simulink model "larix2_tuner"  (R2020b)
settings: Solver=FixedStepDiscrete  StartTime=0.0  StopTime=6  FixedStep=0.002  RelTol=1e-3
PostLoadFcn:
  | load('ThrustTable.mat');
  | init();
values from neighbouring files (symbols this model uses):
  g = 9.810    (= 9.81)    [init.m]
undefined symbols (not defined in the file or in its folder): DiscIntNeverNeededParam
libraries: slpidlib x9, sharedtransform x2, aerolibutil x1
settings Model: Creator=ac114611  LastModifiedBy=wendelin
settings DataIOCC: ExternalInput=getinputstruct(op_hover)  InitialState=getstatestruct(op_hover)  LoadExternalInput=on  LoadInitialState=on  ReturnWorkspaceOutputs=off
settings OptimizationCC: DefaultParameterBehavior=Inlined  EnhancedBackFolding=on  PassReuseOutputArgsAs=Individual arguments  MaxStackSize=64  OptimizeBlockOrder=speed  DifferentSizesBufferReuse=on  EfficientTunableParamExpr=on
settings DebuggingCC: ParameterPrecisionLossMsg=none  ParameterTunabilityLossMsg=error  ArithmeticOperatorsInVariantConditions=warning
settings HardwareCC: ProdBitPerPointer=32  ProdBitPerSizeT=32  ProdBitPerPtrDiffT=32  ProdLargestAtomicInteger=Long  ProdLargestAtomicFloat=Double  ProdWordSize=32  ProdHWDeviceType=ARM Compatible->ARM Cortex  TargetBitPerLong=64  TargetBitPerPointer=64  TargetBitPerSizeT=64  TargetBitPerPtrDiffT=64  TargetLongLongMode=on  TargetIntDivRoundTo=Zero  TargetEndianess=LittleEndian  TargetWordSize=64  TargetHWDeviceType=MATLAB Host  ProdEqTarget=off
settings SFSimCC: SimUseLocalCustomCode=off  MATLABDynamicMemAlloc=off  CustomCodeUndefinedFunction=UseInterfaceOnly
settings RTWCC: Description=Embedded Coder  SystemTargetFile=ert.tlc  GenCodeOnly=on  PackageName=larix2_codegen.zip  TemplateMakefile=ert_default_tmf  RTWUseLocalCustomCode=off  Toolchain=GNU gcc/g++ | gmake (64-bit Linux)  IncludeHyperlinkInReport=on  GenerateCodeMetricsReport=on
settings CodeAppCC: ForceParamTrailComments=on  IgnoreCustomStorageClasses=off  OperatorAnnotations=on  SimulinkDataObjDesc=on  SFDataObjDesc=on  InsertBlockDesc=on
settings ERTTargetCC: TargetLangStandard=C99 (ISO)  InlinedParameterPlacement=NonHierarchical  ERTCustomFileTemplate=example_file_process.tlc

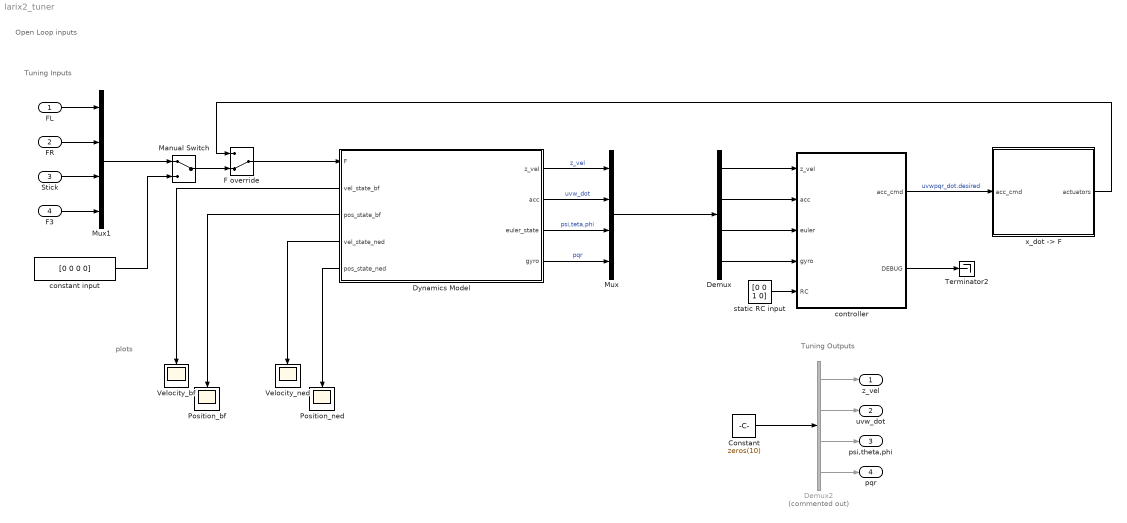
== system larix2_tuner ==
  note: Open Loop inputs
  note: plots
  note: Tuning Inputs
  note: Tuning Outputs
  FL : Inport  PortDimensions=1
  FR : Inport  Port=2
  Stick : Inport  Port=3
  F3 : Inport  Port=4
  Constant : Constant  Value=zeros(10)
  Demux : Demux
  Demux2 : Demux  Commented=on
  Dynamics Model : Subsystem
      settings: PortSchema="{\"entries\":[{\"content\":{\"sides\":[{\"content\":{\"connectorIds\":[\"In1\",\"Out5\",\"Out6\",\"Out7\",\"Out8\"]},\"type\":\"ConnectorPlacement.EquallySpacedRectSide\",\"uuid\":\"7b482eda-451f-4705-a72e-674db1e2ea8f\"},{\"content\":{\"connectorIds\":[\"Out1\",\"Out2\",\"Out3\",\"Out4\"],\"side\":\"RIGHT\"},\"type\":\"ConnectorPlacement.EquallySpacedRectSide\",\"uuid\":\"2344d3e9-2a2c-4bd3-8790-1f9d37abcd4c\"},{\"content\":{\"connectorIds\":[],\"side\":\"TOP\"},\"type\":\"ConnectorPlacement.EquallySpacedRectSide\",\"uuid\":\"13a22bb4-0a82-4477-a366-02f381e5ef07\"},{\"content\":{\"connectorIds\":[],\"side\":\"BOTTOM\"},\"type\":\"ConnectorPlacement.EquallySpacedRectSide\",\"uuid\":\"663825dc-fe4c-484f-87e0-eae3c1c76089\"},{\"content\":{\"connectorIds\":[],\"side\":\"HIDDEN\"},\"type\":\"ConnectorPlacement.EquallySpacedRectSide\",\"uuid\":\"0874c0d1-0ac2-489a-adcf-241d9ac40396\"}]},\"type\":\"ConnectorPlacement.EquallySpacedConnector\",\"uuid\":\"4f633129-49ae-43ab-aa97-bf1abe451306\"}],\"packageUris\":[\"http://schema.mathworks.com/mf0/Connector/R2020b\"],\"version\":\"1.0\"}"
  F override : ManualSwitch  CurrentSetting=0
  Manual Switch : ManualSwitch
  Mux : Mux
  Mux1 : Mux
  Position_bf : Scope
  Position_ned : Scope
  Terminator2 : Terminator
  Velocity_bf : Scope
  Velocity_ned : Scope
  constant input : Constant  Value=[0 0 0 0]
  controller : Subsystem
  static RC input : Constant  Value=[0 0 1 0]
  "x_dot -> F" : Subsystem
  z_vel : Outport  PortDimensions=1
  uvw_dot : Outport  Port=2  PortDimensions=3
  psi,theta,phi : Outport  Port=3  PortDimensions=3
  pqr : Outport  Port=4  PortDimensions=3
  wires:
  Dynamics Model/4(gyro) -> Mux/4  "pqr"
  controller/2(DEBUG) -> Terminator2/1
  controller/1(acc_cmd) -> "x_dot -> F"/1(acc_cmd)  "uvwpqr_dot.desired"
  "x_dot -> F"/1(actuators) -> F override/1
  Dynamics Model/2(acc) -> Mux/2  "uvw_dot"
  Dynamics Model/1(z_vel) -> Mux/1  "z_vel"
  Dynamics Model/3(euler_state) -> Mux/3  "psi,teta,phi"
  Dynamics Model/6(pos_state_bf) -> Position_bf/1
  Dynamics Model/5(vel_state_bf) -> Velocity_bf/1
  static RC input/1 -> controller/5(RC)
  F override/1 -> Dynamics Model/1(F)
  Demux/1 -> controller/1(z_vel)
  Demux/2 -> controller/2(acc)
  Demux/3 -> controller/3(euler)
  Demux/4 -> controller/4(gyro)
  Mux/1 -> Demux/1
  Constant/1 -> Demux2/1
  Demux2/1 -> z_vel/1
  Demux2/2 -> uvw_dot/1
  Demux2/4 -> pqr/1
  Demux2/3 -> psi,theta,phi/1
  FL/1 -> Mux1/1
  FR/1 -> Mux1/2
  Stick/1 -> Mux1/3
  F3/1 -> Mux1/4
  Mux1/1 -> Manual Switch/1
  Dynamics Model/7(vel_state_ned) -> Velocity_ned/1
  Dynamics Model/8(pos_state_ned) -> Position_ned/1
  Manual Switch/1 -> F override/2
  constant input/1 -> Manual Switch/2

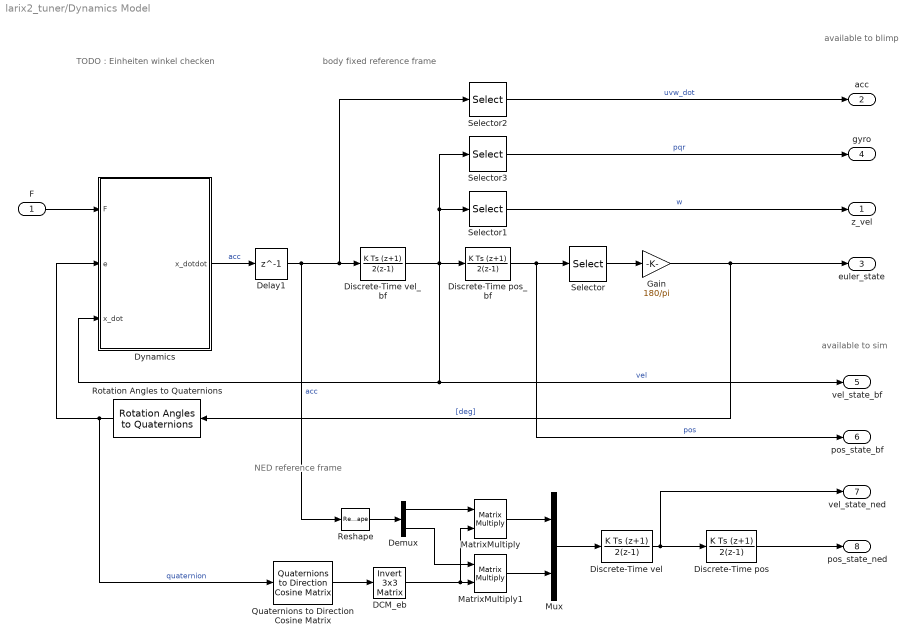
== system larix2_tuner/Dynamics Model ==
  note: NED reference frame
  note: body fixed reference frame
  note: TODO : Einheiten winkel checken
  note: available
      | to sim
  note: available
      | to blimp
  F : Inport
  DCM_eb : aerolibutil/Invert  3x3 Matrix
  Delay1 : Delay  DelayLength=1
  Demux : Demux  Outputs=2
  Discrete-Time pos : DiscreteIntegrator  IntegratorMethod=Integration: Trapezoidal  SampleTime=-1  StateName=position_ned  ICPrevOutput=DiscIntNeverNeededParam  ICPrevScaledInput=DiscIntNeverNeededParam
  Discrete-Time pos_bf : DiscreteIntegrator  IntegratorMethod=Integration: Trapezoidal  SampleTime=-1  StateName=position  ICPrevOutput=DiscIntNeverNeededParam  ICPrevScaledInput=DiscIntNeverNeededParam
  Discrete-Time vel : DiscreteIntegrator  IntegratorMethod=Integration: Trapezoidal  SampleTime=-1  StateName=velocity_ned  ICPrevOutput=DiscIntNeverNeededParam  ICPrevScaledInput=DiscIntNeverNeededParam
  Discrete-Time vel_bf : DiscreteIntegrator  IntegratorMethod=Integration: Trapezoidal  SampleTime=-1  StateName=velocity  ICPrevOutput=DiscIntNeverNeededParam  ICPrevScaledInput=DiscIntNeverNeededParam
  Dynamics : MATLAB Function  TreatAsAtomicUnit=on
  Gain : Gain  Gain=180/pi
  MatrixMultiply : Product  Inputs=**  Multiplication=Matrix(*)
  MatrixMultiply1 : Product  Inputs=**  Multiplication=Matrix(*)
  Mux : Mux  Inputs=2
  Quaternions to Direction Cosine Matrix : sharedtransform/Quaternions to  Direction Cosine Matrix  aMode=aMode
      settings: SourceProductBaseCode=AE,PW,MT,UV,VE,VP
  Reshape : Reshape  OutputDimensionality=Customize  OutputDimensions=[1,6]
  Rotation Angles to Quaternions : sharedtransform/Rotation Angles to Quaternions  rotationOrder=ZYX  aMode=aMode
      settings: SourceProductBaseCode=AE,PW,MT,UV,VE,VP
  Selector : Selector  InputPortWidth=6  IndexOptions=Index vector (dialog)  Indices=[4 5 6]  OutputSizes=1
  Selector1 : Selector  InputPortWidth=6  IndexOptions=Index vector (dialog)  Indices=[3]  OutputSizes=1
  Selector2 : Selector  InputPortWidth=6  IndexOptions=Index vector (dialog)  Indices=[1 2 3]  OutputSizes=1
  Selector3 : Selector  InputPortWidth=6  IndexOptions=Index vector (dialog)  Indices=[4 5 6]  OutputSizes=1
  z_vel : Outport  OutDataTypeStr=double
  acc : Outport  Port=2  OutDataTypeStr=double
  euler_state : Outport  Port=3  OutDataTypeStr=double
  gyro : Outport  Port=4  OutDataTypeStr=double
  vel_state_bf : Outport  Port=5  OutDataTypeStr=double
  pos_state_bf : Outport  Port=6  OutDataTypeStr=double
  vel_state_ned : Outport  Port=7
  pos_state_ned : Outport  Port=8
  wires:
  Discrete-Time pos_bf/1 -> pos_state_bf/1, Selector/1  "pos"
  Discrete-Time vel_bf/1 -> Dynamics/3(x_dot), vel_state_bf/1, Discrete-Time pos_bf/1, Selector3/1, Selector1/1  "vel"
  F/1 -> Dynamics/1(F)
  Rotation Angles to Quaternions/1 -> Quaternions to Direction Cosine Matrix/1, Dynamics/2(e)  "quaternion"
  Dynamics/1(x_dotdot) -> Delay1/1  "acc"
  Selector1/1 -> z_vel/1  "w"
  Selector2/1 -> acc/1  "uvw_dot"
  Delay1/1 -> Discrete-Time vel_bf/1, Selector2/1, Reshape/1  "acc"
  Selector/1 -> Gain/1
  Gain/1 -> Rotation Angles to Quaternions/1, euler_state/1  "[deg]"
  Selector3/1 -> gyro/1  "pqr"
  Quaternions to Direction Cosine Matrix/1 -> DCM_eb/1
  DCM_eb/1 -> MatrixMultiply/2, MatrixMultiply1/2
  MatrixMultiply/1 -> Mux/1
  Discrete-Time vel/1 -> Discrete-Time pos/1, vel_state_ned/1
  Discrete-Time pos/1 -> pos_state_ned/1
  Demux/1 -> MatrixMultiply/1
  Demux/2 -> MatrixMultiply1/1
  MatrixMultiply1/1 -> Mux/2
  Mux/1 -> Discrete-Time vel/1
  Reshape/1 -> Demux/1

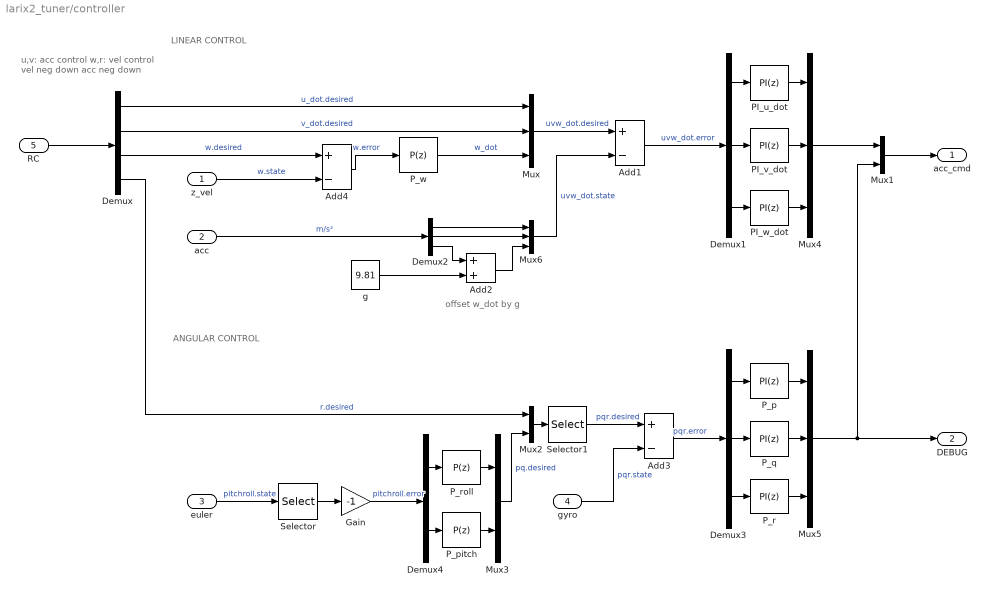
== system larix2_tuner/controller ==
  note: offset w_dot by g
  note: u,v: acc control
      | w,r: vel control
      |
      | vel neg down
      | acc neg down
  note: LINEAR CONTROL
  note: ANGULAR CONTROL
  z_vel : Inport  PortDimensions=1
  acc : Inport  Port=2  PortDimensions=3
  euler : Inport  Port=3  PortDimensions=3
  gyro : Inport  Port=4  PortDimensions=3
  RC : Inport  Port=5
  Add1 : Sum  Inputs=+-
  Add2 : Sum
  Add3 : Sum  Inputs=+-
  Add4 : Sum  Inputs=+-
  Demux : Demux
  Demux1 : Demux  Outputs=3
  Demux2 : Demux  Outputs=3
  Demux3 : Demux  Outputs=3
  Demux4 : Demux  Outputs=2
  Gain : Gain  Gain=-1
  Mux{,4..6} (4 alike) : Mux  Inputs=3
  Mux1 : Mux  Inputs=2
  Mux2 : Mux  Inputs=2
  Mux3 : Mux  Inputs=2
  PI_u_dot : slpidlib/PID Controller  Controller=PI  Form=Parallel  TimeDomain=Discrete-time  UseExternalTs=off  SampleTime=-1  IntegratorMethod=Trapezoidal  FilterMethod=Forward Euler  ControllerParametersSource=internal  P=0.5  I=0.2  D=0  UseFilter=on  N=100  TunerSelectOption=Transfer Function Based (PID Tuner App)  InitialConditionSource=internal  InitialConditionForIntegrator=0  InitialConditionForFilter=0  DifferentiatorICPrevScaledInput=0  ExternalReset=none  TrackingMode=off  Kt=1  LimitOutput=off  SatLimitsSource=internal  UpperSaturationLimit=0.4*g  LowerSaturationLimit=-0.4*g  LinearizeAsGain=off  AntiWindupMode=none  Kb=1  POutMin=[]  POutMax=[]  IOutMin=[]  IOutMax=[]  DOutMin=[]  DOutMax=[]  NOutMin=[]  NOutMax=[]  SumOutMin=[]  SumOutMax=[]  SaturationOutMin=[]  SaturationOutMax=[]  PParamMin=[]  PParamMax=[]  IParamMin=[]  IParamMax=[]  DParamMin=[]  DParamMax=[]  NParamMin=[]  NParamMax=[]  KbParamMin=[]  KbParamMax=[]  KtParamMin=[]  KtParamMax=[]  KbOutMin=[]  KbOutMax=[]  KtOutMin=[]  KtOutMax=[]  IntegratorOutMin=[]  IntegratorOutMax=[]  FilterOutMin=[]  FilterOutMax=[]  SumI1OutMin=[]  SumI1OutMax=[]  SumI2OutMin=[]  SumI2OutMax=[]  SumI3OutMin=[]  SumI3OutMax=[]  SumI4OutMin=[]  SumI4OutMax=[]  SumDOutMin=[]  SumDOutMax=[]  DifferentiatorOutMin=[]  DifferentiatorOutMax=[]  FilterDiffOutCoefMin=[]  FilterDiffOutCoefMax=[]  ReciprocalOutMin=[]  ReciprocalOutMax=[]  SumDenOutMin=[]  SumDenOutMax=[]  SumNumOutMin=[]  SumNumOutMax=[]  DivideOutMin=[]  DivideOutMax=[]  UdiffTsProdOutMin=[]  UdiffTsProdOutMax=[]  NTsProdOutMin=[]  NTsProdOutMax=[]  UintegralTsProdOutMin=[]  UintegralTsProdOutMax=[]  UngainTsProdOutMin=[]  UngainTsProdOutMax=[]  IntegratorContinuousStateAttributes=''  IntegratorStateMustResolveToSignalObject=off  IntegratorRTWStateStorageClass=Auto  FilterContinuousStateAttributes=''  FilterStateMustResolveToSignalObject=off  FilterRTWStateStorageClass=Auto  ParallelPVariant=InternalParameters  IdealPVariant=Disabled  IVariant=InternalParameters  DVariant=Disabled  IntegratorVariant=Discrete  SatVariant=Disabled  AWVariant=Passthrough  PCopyVariant=Disabled  TRVariant=Disabled  FdbkBlocksVariant=Forward  IdealPFdbkVariant=Disabled  SatFdbkVariant=Disabled  DerivativeFilterVariant=Disabled  NVariant=Disabled  NCopyVariant=Disabled_SignalSpec  FilterICVariant=Disabled  IntegratorICVariant=InternalICs  ExternalResetVariant=Disabled  TRSumVariant=Passthrough  SumFdbkVariant=Disabled  SumVariant=Sum_PI  TsampFilterVariant=InternalTs  TsampNgainVariant=Passthrough  TsampIntegralVariant=Passthrough  ExternalSaturationOutDataTypeStr=Inherit: Same as second input
  PI_v_dot : slpidlib/PID Controller  Controller=PI  Form=Parallel  TimeDomain=Discrete-time  UseExternalTs=off  SampleTime=-1  IntegratorMethod=Forward Euler  FilterMethod=Forward Euler  ControllerParametersSource=internal  P=0.6  I=0  D=0  UseFilter=on  N=100  TunerSelectOption=Transfer Function Based (PID Tuner App)  InitialConditionSource=internal  InitialConditionForIntegrator=0  InitialConditionForFilter=0  DifferentiatorICPrevScaledInput=0  ExternalReset=none  TrackingMode=off  Kt=1  LimitOutput=off  SatLimitsSource=internal  UpperSaturationLimit=inf  LowerSaturationLimit=-inf  LinearizeAsGain=off  AntiWindupMode=none  Kb=1  POutMin=[]  POutMax=[]  IOutMin=[]  IOutMax=[]  DOutMin=[]  DOutMax=[]  NOutMin=[]  NOutMax=[]  SumOutMin=[]  SumOutMax=[]  SaturationOutMin=[]  SaturationOutMax=[]  PParamMin=[]  PParamMax=[]  IParamMin=[]  IParamMax=[]  DParamMin=[]  DParamMax=[]  NParamMin=[]  NParamMax=[]  KbParamMin=[]  KbParamMax=[]  KtParamMin=[]  KtParamMax=[]  KbOutMin=[]  KbOutMax=[]  KtOutMin=[]  KtOutMax=[]  IntegratorOutMin=[]  IntegratorOutMax=[]  FilterOutMin=[]  FilterOutMax=[]  SumI1OutMin=[]  SumI1OutMax=[]  SumI2OutMin=[]  SumI2OutMax=[]  SumI3OutMin=[]  SumI3OutMax=[]  SumI4OutMin=[]  SumI4OutMax=[]  SumDOutMin=[]  SumDOutMax=[]  DifferentiatorOutMin=[]  DifferentiatorOutMax=[]  FilterDiffOutCoefMin=[]  FilterDiffOutCoefMax=[]  ReciprocalOutMin=[]  ReciprocalOutMax=[]  SumDenOutMin=[]  SumDenOutMax=[]  SumNumOutMin=[]  SumNumOutMax=[]  DivideOutMin=[]  DivideOutMax=[]  UdiffTsProdOutMin=[]  UdiffTsProdOutMax=[]  NTsProdOutMin=[]  NTsProdOutMax=[]  UintegralTsProdOutMin=[]  UintegralTsProdOutMax=[]  UngainTsProdOutMin=[]  UngainTsProdOutMax=[]  IntegratorContinuousStateAttributes=''  IntegratorStateMustResolveToSignalObject=off  IntegratorRTWStateStorageClass=Auto  FilterContinuousStateAttributes=''  FilterStateMustResolveToSignalObject=off  FilterRTWStateStorageClass=Auto  ParallelPVariant=InternalParameters  IdealPVariant=Disabled  IVariant=InternalParameters  DVariant=Disabled  IntegratorVariant=Discrete  SatVariant=Disabled  AWVariant=Passthrough  PCopyVariant=Disabled  TRVariant=Disabled  FdbkBlocksVariant=Forward  IdealPFdbkVariant=Disabled  SatFdbkVariant=Disabled  DerivativeFilterVariant=Disabled  NVariant=Disabled  NCopyVariant=Disabled_SignalSpec  FilterICVariant=Disabled  IntegratorICVariant=InternalICs  ExternalResetVariant=Disabled  TRSumVariant=Passthrough  SumFdbkVariant=Disabled  SumVariant=Sum_PI  TsampFilterVariant=InternalTs  TsampNgainVariant=Passthrough  TsampIntegralVariant=Passthrough  ExternalSaturationOutDataTypeStr=Inherit: Same as second input
  PI_w_dot : slpidlib/PID Controller  Controller=PI  Form=Parallel  TimeDomain=Discrete-time  UseExternalTs=off  SampleTime=-1  IntegratorMethod=Forward Euler  FilterMethod=Forward Euler  ControllerParametersSource=internal  P=1.2  I=0  D=0  UseFilter=on  N=100  TunerSelectOption=Transfer Function Based (PID Tuner App)  InitialConditionSource=internal  InitialConditionForIntegrator=0  InitialConditionForFilter=0  DifferentiatorICPrevScaledInput=0  ExternalReset=none  TrackingMode=off  Kt=1  LimitOutput=off  SatLimitsSource=internal  UpperSaturationLimit=inf  LowerSaturationLimit=0  LinearizeAsGain=off  AntiWindupMode=none  Kb=1  POutMin=[]  POutMax=[]  IOutMin=[]  IOutMax=[]  DOutMin=[]  DOutMax=[]  NOutMin=[]  NOutMax=[]  SumOutMin=[]  SumOutMax=[]  SaturationOutMin=[]  SaturationOutMax=[]  PParamMin=[]  PParamMax=[]  IParamMin=[]  IParamMax=[]  DParamMin=[]  DParamMax=[]  NParamMin=[]  NParamMax=[]  KbParamMin=[]  KbParamMax=[]  KtParamMin=[]  KtParamMax=[]  KbOutMin=[]  KbOutMax=[]  KtOutMin=[]  KtOutMax=[]  IntegratorOutMin=[]  IntegratorOutMax=[]  FilterOutMin=[]  FilterOutMax=[]  SumI1OutMin=[]  SumI1OutMax=[]  SumI2OutMin=[]  SumI2OutMax=[]  SumI3OutMin=[]  SumI3OutMax=[]  SumI4OutMin=[]  SumI4OutMax=[]  SumDOutMin=[]  SumDOutMax=[]  DifferentiatorOutMin=[]  DifferentiatorOutMax=[]  FilterDiffOutCoefMin=[]  FilterDiffOutCoefMax=[]  ReciprocalOutMin=[]  ReciprocalOutMax=[]  SumDenOutMin=[]  SumDenOutMax=[]  SumNumOutMin=[]  SumNumOutMax=[]  DivideOutMin=[]  DivideOutMax=[]  UdiffTsProdOutMin=[]  UdiffTsProdOutMax=[]  NTsProdOutMin=[]  NTsProdOutMax=[]  UintegralTsProdOutMin=[]  UintegralTsProdOutMax=[]  UngainTsProdOutMin=[]  UngainTsProdOutMax=[]  IntegratorContinuousStateAttributes=''  IntegratorStateMustResolveToSignalObject=off  IntegratorRTWStateStorageClass=Auto  FilterContinuousStateAttributes=''  FilterStateMustResolveToSignalObject=off  FilterRTWStateStorageClass=Auto  ParallelPVariant=InternalParameters  IdealPVariant=Disabled  IVariant=InternalParameters  DVariant=Disabled  IntegratorVariant=Discrete  SatVariant=Disabled  AWVariant=Passthrough  PCopyVariant=Disabled  TRVariant=Disabled  FdbkBlocksVariant=Forward  IdealPFdbkVariant=Disabled  SatFdbkVariant=Disabled  DerivativeFilterVariant=Disabled  NVariant=Disabled  NCopyVariant=Disabled_SignalSpec  FilterICVariant=Disabled  IntegratorICVariant=InternalICs  ExternalResetVariant=Disabled  TRSumVariant=Passthrough  SumFdbkVariant=Disabled  SumVariant=Sum_PI  TsampFilterVariant=InternalTs  TsampNgainVariant=Passthrough  TsampIntegralVariant=Passthrough  ExternalSaturationOutDataTypeStr=Inherit: Same as second input
  P_p : slpidlib/PID Controller  Controller=PI  Form=Parallel  TimeDomain=Discrete-time  UseExternalTs=off  SampleTime=-1  IntegratorMethod=Forward Euler  FilterMethod=Forward Euler  ControllerParametersSource=internal  P=0.3  I=0  D=0  UseFilter=on  N=100  TunerSelectOption=Transfer Function Based (PID Tuner App)  InitialConditionSource=internal  InitialConditionForIntegrator=0  InitialConditionForFilter=0  DifferentiatorICPrevScaledInput=0  ExternalReset=none  TrackingMode=off  Kt=1  LimitOutput=off  SatLimitsSource=internal  UpperSaturationLimit=inf  LowerSaturationLimit=-inf  LinearizeAsGain=on  AntiWindupMode=none  Kb=1  POutMin=[]  POutMax=[]  IOutMin=[]  IOutMax=[]  DOutMin=[]  DOutMax=[]  NOutMin=[]  NOutMax=[]  SumOutMin=[]  SumOutMax=[]  SaturationOutMin=[]  SaturationOutMax=[]  PParamMin=[]  PParamMax=[]  IParamMin=[]  IParamMax=[]  DParamMin=[]  DParamMax=[]  NParamMin=[]  NParamMax=[]  KbParamMin=[]  KbParamMax=[]  KtParamMin=[]  KtParamMax=[]  KbOutMin=[]  KbOutMax=[]  KtOutMin=[]  KtOutMax=[]  IntegratorOutMin=[]  IntegratorOutMax=[]  FilterOutMin=[]  FilterOutMax=[]  SumI1OutMin=[]  SumI1OutMax=[]  SumI2OutMin=[]  SumI2OutMax=[]  SumI3OutMin=[]  SumI3OutMax=[]  SumI4OutMin=[]  SumI4OutMax=[]  SumDOutMin=[]  SumDOutMax=[]  DifferentiatorOutMin=[]  DifferentiatorOutMax=[]  FilterDiffOutCoefMin=[]  FilterDiffOutCoefMax=[]  ReciprocalOutMin=[]  ReciprocalOutMax=[]  SumDenOutMin=[]  SumDenOutMax=[]  SumNumOutMin=[]  SumNumOutMax=[]  DivideOutMin=[]  DivideOutMax=[]  UdiffTsProdOutMin=[]  UdiffTsProdOutMax=[]  NTsProdOutMin=[]  NTsProdOutMax=[]  UintegralTsProdOutMin=[]  UintegralTsProdOutMax=[]  UngainTsProdOutMin=[]  UngainTsProdOutMax=[]  IntegratorContinuousStateAttributes=''  IntegratorStateMustResolveToSignalObject=off  IntegratorRTWStateStorageClass=Auto  FilterContinuousStateAttributes=''  FilterStateMustResolveToSignalObject=off  FilterRTWStateStorageClass=Auto  ParallelPVariant=InternalParameters  IdealPVariant=Disabled  IVariant=InternalParameters  DVariant=Disabled  IntegratorVariant=Discrete  SatVariant=Disabled  AWVariant=Passthrough  PCopyVariant=Disabled  TRVariant=Disabled  FdbkBlocksVariant=Forward  IdealPFdbkVariant=Disabled  SatFdbkVariant=Disabled  DerivativeFilterVariant=Disabled  NVariant=Disabled  NCopyVariant=Disabled_SignalSpec  FilterICVariant=Disabled  IntegratorICVariant=InternalICs  ExternalResetVariant=Disabled  TRSumVariant=Passthrough  SumFdbkVariant=Disabled  SumVariant=Sum_PI  TsampFilterVariant=InternalTs  TsampNgainVariant=Passthrough  TsampIntegralVariant=Passthrough  ExternalSaturationOutDataTypeStr=Inherit: Same as second input
  P_pitch : slpidlib/PID Controller  Controller=P  Form=Parallel  TimeDomain=Discrete-time  UseExternalTs=off  SampleTime=-1  IntegratorMethod=Forward Euler  FilterMethod=Forward Euler  ControllerParametersSource=internal  P=0.3  I=0  D=0  UseFilter=on  N=100  TunerSelectOption=Transfer Function Based (PID Tuner App)  InitialConditionSource=internal  InitialConditionForIntegrator=0  InitialConditionForFilter=0  DifferentiatorICPrevScaledInput=0  ExternalReset=none  TrackingMode=off  Kt=1  LimitOutput=off  SatLimitsSource=internal  UpperSaturationLimit=inf  LowerSaturationLimit=-inf  LinearizeAsGain=on  AntiWindupMode=none  Kb=1  POutMin=[]  POutMax=[]  IOutMin=[]  IOutMax=[]  DOutMin=[]  DOutMax=[]  NOutMin=[]  NOutMax=[]  SumOutMin=[]  SumOutMax=[]  SaturationOutMin=[]  SaturationOutMax=[]  PParamMin=[]  PParamMax=[]  IParamMin=[]  IParamMax=[]  DParamMin=[]  DParamMax=[]  NParamMin=[]  NParamMax=[]  KbParamMin=[]  KbParamMax=[]  KtParamMin=[]  KtParamMax=[]  KbOutMin=[]  KbOutMax=[]  KtOutMin=[]  KtOutMax=[]  IntegratorOutMin=[]  IntegratorOutMax=[]  FilterOutMin=[]  FilterOutMax=[]  SumI1OutMin=[]  SumI1OutMax=[]  SumI2OutMin=[]  SumI2OutMax=[]  SumI3OutMin=[]  SumI3OutMax=[]  SumI4OutMin=[]  SumI4OutMax=[]  SumDOutMin=[]  SumDOutMax=[]  DifferentiatorOutMin=[]  DifferentiatorOutMax=[]  FilterDiffOutCoefMin=[]  FilterDiffOutCoefMax=[]  ReciprocalOutMin=[]  ReciprocalOutMax=[]  SumDenOutMin=[]  SumDenOutMax=[]  SumNumOutMin=[]  SumNumOutMax=[]  DivideOutMin=[]  DivideOutMax=[]  UdiffTsProdOutMin=[]  UdiffTsProdOutMax=[]  NTsProdOutMin=[]  NTsProdOutMax=[]  UintegralTsProdOutMin=[]  UintegralTsProdOutMax=[]  UngainTsProdOutMin=[]  UngainTsProdOutMax=[]  IntegratorContinuousStateAttributes=''  IntegratorStateMustResolveToSignalObject=off  IntegratorRTWStateStorageClass=Auto  FilterContinuousStateAttributes=''  FilterStateMustResolveToSignalObject=off  FilterRTWStateStorageClass=Auto  ParallelPVariant=InternalParameters  IdealPVariant=Disabled  IVariant=Disabled  DVariant=Disabled  IntegratorVariant=Disabled  SatVariant=Disabled  AWVariant=Disabled  PCopyVariant=Disabled  TRVariant=Disabled  FdbkBlocksVariant=Forward  IdealPFdbkVariant=Disabled  SatFdbkVariant=Disabled  DerivativeFilterVariant=Disabled  NVariant=Disabled  NCopyVariant=Disabled_SignalSpec  FilterICVariant=Disabled  IntegratorICVariant=Disabled  ExternalResetVariant=Disabled  TRSumVariant=Passthrough  SumFdbkVariant=Disabled  SumVariant=Passthrough_P  TsampFilterVariant=InternalTs  TsampNgainVariant=Passthrough  TsampIntegralVariant=Disabled_SignalSpec  ExternalSaturationOutDataTypeStr=Inherit: Same as second input
  P_q : slpidlib/PID Controller  Controller=PI  Form=Parallel  TimeDomain=Discrete-time  UseExternalTs=off  SampleTime=-1  IntegratorMethod=Forward Euler  FilterMethod=Forward Euler  ControllerParametersSource=internal  P=1  I=0  D=0  UseFilter=on  N=100  TunerSelectOption=Transfer Function Based (PID Tuner App)  InitialConditionSource=internal  InitialConditionForIntegrator=0  InitialConditionForFilter=0  DifferentiatorICPrevScaledInput=0  ExternalReset=none  TrackingMode=off  Kt=1  LimitOutput=off  SatLimitsSource=internal  UpperSaturationLimit=inf  LowerSaturationLimit=-inf  LinearizeAsGain=on  AntiWindupMode=none  Kb=1  POutMin=[]  POutMax=[]  IOutMin=[]  IOutMax=[]  DOutMin=[]  DOutMax=[]  NOutMin=[]  NOutMax=[]  SumOutMin=[]  SumOutMax=[]  SaturationOutMin=[]  SaturationOutMax=[]  PParamMin=[]  PParamMax=[]  IParamMin=[]  IParamMax=[]  DParamMin=[]  DParamMax=[]  NParamMin=[]  NParamMax=[]  KbParamMin=[]  KbParamMax=[]  KtParamMin=[]  KtParamMax=[]  KbOutMin=[]  KbOutMax=[]  KtOutMin=[]  KtOutMax=[]  IntegratorOutMin=[]  IntegratorOutMax=[]  FilterOutMin=[]  FilterOutMax=[]  SumI1OutMin=[]  SumI1OutMax=[]  SumI2OutMin=[]  SumI2OutMax=[]  SumI3OutMin=[]  SumI3OutMax=[]  SumI4OutMin=[]  SumI4OutMax=[]  SumDOutMin=[]  SumDOutMax=[]  DifferentiatorOutMin=[]  DifferentiatorOutMax=[]  FilterDiffOutCoefMin=[]  FilterDiffOutCoefMax=[]  ReciprocalOutMin=[]  ReciprocalOutMax=[]  SumDenOutMin=[]  SumDenOutMax=[]  SumNumOutMin=[]  SumNumOutMax=[]  DivideOutMin=[]  DivideOutMax=[]  UdiffTsProdOutMin=[]  UdiffTsProdOutMax=[]  NTsProdOutMin=[]  NTsProdOutMax=[]  UintegralTsProdOutMin=[]  UintegralTsProdOutMax=[]  UngainTsProdOutMin=[]  UngainTsProdOutMax=[]  IntegratorContinuousStateAttributes=''  IntegratorStateMustResolveToSignalObject=off  IntegratorRTWStateStorageClass=Auto  FilterContinuousStateAttributes=''  FilterStateMustResolveToSignalObject=off  FilterRTWStateStorageClass=Auto  ParallelPVariant=InternalParameters  IdealPVariant=Disabled  IVariant=InternalParameters  DVariant=Disabled  IntegratorVariant=Discrete  SatVariant=Disabled  AWVariant=Passthrough  PCopyVariant=Disabled  TRVariant=Disabled  FdbkBlocksVariant=Forward  IdealPFdbkVariant=Disabled  SatFdbkVariant=Disabled  DerivativeFilterVariant=Disabled  NVariant=Disabled  NCopyVariant=Disabled_SignalSpec  FilterICVariant=Disabled  IntegratorICVariant=InternalICs  ExternalResetVariant=Disabled  TRSumVariant=Passthrough  SumFdbkVariant=Disabled  SumVariant=Sum_PI  TsampFilterVariant=InternalTs  TsampNgainVariant=Passthrough  TsampIntegralVariant=Passthrough  ExternalSaturationOutDataTypeStr=Inherit: Same as second input
  P_r : slpidlib/PID Controller  Controller=PI  Form=Parallel  TimeDomain=Discrete-time  UseExternalTs=off  SampleTime=-1  IntegratorMethod=Forward Euler  FilterMethod=Forward Euler  ControllerParametersSource=internal  P=0.8  I=0  D=0  UseFilter=on  N=100  TunerSelectOption=Transfer Function Based (PID Tuner App)  InitialConditionSource=internal  InitialConditionForIntegrator=0  InitialConditionForFilter=0  DifferentiatorICPrevScaledInput=0  ExternalReset=none  TrackingMode=off  Kt=1  LimitOutput=off  SatLimitsSource=internal  UpperSaturationLimit=inf  LowerSaturationLimit=-inf  LinearizeAsGain=on  AntiWindupMode=none  Kb=1  POutMin=[]  POutMax=[]  IOutMin=[]  IOutMax=[]  DOutMin=[]  DOutMax=[]  NOutMin=[]  NOutMax=[]  SumOutMin=[]  SumOutMax=[]  SaturationOutMin=[]  SaturationOutMax=[]  PParamMin=[]  PParamMax=[]  IParamMin=[]  IParamMax=[]  DParamMin=[]  DParamMax=[]  NParamMin=[]  NParamMax=[]  KbParamMin=[]  KbParamMax=[]  KtParamMin=[]  KtParamMax=[]  KbOutMin=[]  KbOutMax=[]  KtOutMin=[]  KtOutMax=[]  IntegratorOutMin=[]  IntegratorOutMax=[]  FilterOutMin=[]  FilterOutMax=[]  SumI1OutMin=[]  SumI1OutMax=[]  SumI2OutMin=[]  SumI2OutMax=[]  SumI3OutMin=[]  SumI3OutMax=[]  SumI4OutMin=[]  SumI4OutMax=[]  SumDOutMin=[]  SumDOutMax=[]  DifferentiatorOutMin=[]  DifferentiatorOutMax=[]  FilterDiffOutCoefMin=[]  FilterDiffOutCoefMax=[]  ReciprocalOutMin=[]  ReciprocalOutMax=[]  SumDenOutMin=[]  SumDenOutMax=[]  SumNumOutMin=[]  SumNumOutMax=[]  DivideOutMin=[]  DivideOutMax=[]  UdiffTsProdOutMin=[]  UdiffTsProdOutMax=[]  NTsProdOutMin=[]  NTsProdOutMax=[]  UintegralTsProdOutMin=[]  UintegralTsProdOutMax=[]  UngainTsProdOutMin=[]  UngainTsProdOutMax=[]  IntegratorContinuousStateAttributes=''  IntegratorStateMustResolveToSignalObject=off  IntegratorRTWStateStorageClass=Auto  FilterContinuousStateAttributes=''  FilterStateMustResolveToSignalObject=off  FilterRTWStateStorageClass=Auto  ParallelPVariant=InternalParameters  IdealPVariant=Disabled  IVariant=InternalParameters  DVariant=Disabled  IntegratorVariant=Discrete  SatVariant=Disabled  AWVariant=Passthrough  PCopyVariant=Disabled  TRVariant=Disabled  FdbkBlocksVariant=Forward  IdealPFdbkVariant=Disabled  SatFdbkVariant=Disabled  DerivativeFilterVariant=Disabled  NVariant=Disabled  NCopyVariant=Disabled_SignalSpec  FilterICVariant=Disabled  IntegratorICVariant=InternalICs  ExternalResetVariant=Disabled  TRSumVariant=Passthrough  SumFdbkVariant=Disabled  SumVariant=Sum_PI  TsampFilterVariant=InternalTs  TsampNgainVariant=Passthrough  TsampIntegralVariant=Passthrough  ExternalSaturationOutDataTypeStr=Inherit: Same as second input
  P_roll : slpidlib/PID Controller  Controller=P  Form=Parallel  TimeDomain=Discrete-time  UseExternalTs=off  SampleTime=-1  IntegratorMethod=Forward Euler  FilterMethod=Forward Euler  ControllerParametersSource=internal  P=0.3  I=0  D=0  UseFilter=on  N=100  TunerSelectOption=Transfer Function Based (PID Tuner App)  InitialConditionSource=internal  InitialConditionForIntegrator=0  InitialConditionForFilter=0  DifferentiatorICPrevScaledInput=0  ExternalReset=none  TrackingMode=off  Kt=1  LimitOutput=off  SatLimitsSource=internal  UpperSaturationLimit=inf  LowerSaturationLimit=-inf  LinearizeAsGain=on  AntiWindupMode=none  Kb=1  POutMin=[]  POutMax=[]  IOutMin=[]  IOutMax=[]  DOutMin=[]  DOutMax=[]  NOutMin=[]  NOutMax=[]  SumOutMin=[]  SumOutMax=[]  SaturationOutMin=[]  SaturationOutMax=[]  PParamMin=[]  PParamMax=[]  IParamMin=[]  IParamMax=[]  DParamMin=[]  DParamMax=[]  NParamMin=[]  NParamMax=[]  KbParamMin=[]  KbParamMax=[]  KtParamMin=[]  KtParamMax=[]  KbOutMin=[]  KbOutMax=[]  KtOutMin=[]  KtOutMax=[]  IntegratorOutMin=[]  IntegratorOutMax=[]  FilterOutMin=[]  FilterOutMax=[]  SumI1OutMin=[]  SumI1OutMax=[]  SumI2OutMin=[]  SumI2OutMax=[]  SumI3OutMin=[]  SumI3OutMax=[]  SumI4OutMin=[]  SumI4OutMax=[]  SumDOutMin=[]  SumDOutMax=[]  DifferentiatorOutMin=[]  DifferentiatorOutMax=[]  FilterDiffOutCoefMin=[]  FilterDiffOutCoefMax=[]  ReciprocalOutMin=[]  ReciprocalOutMax=[]  SumDenOutMin=[]  SumDenOutMax=[]  SumNumOutMin=[]  SumNumOutMax=[]  DivideOutMin=[]  DivideOutMax=[]  UdiffTsProdOutMin=[]  UdiffTsProdOutMax=[]  NTsProdOutMin=[]  NTsProdOutMax=[]  UintegralTsProdOutMin=[]  UintegralTsProdOutMax=[]  UngainTsProdOutMin=[]  UngainTsProdOutMax=[]  IntegratorContinuousStateAttributes=''  IntegratorStateMustResolveToSignalObject=off  IntegratorRTWStateStorageClass=Auto  FilterContinuousStateAttributes=''  FilterStateMustResolveToSignalObject=off  FilterRTWStateStorageClass=Auto  ParallelPVariant=InternalParameters  IdealPVariant=Disabled  IVariant=Disabled  DVariant=Disabled  IntegratorVariant=Disabled  SatVariant=Disabled  AWVariant=Disabled  PCopyVariant=Disabled  TRVariant=Disabled  FdbkBlocksVariant=Forward  IdealPFdbkVariant=Disabled  SatFdbkVariant=Disabled  DerivativeFilterVariant=Disabled  NVariant=Disabled  NCopyVariant=Disabled_SignalSpec  FilterICVariant=Disabled  IntegratorICVariant=Disabled  ExternalResetVariant=Disabled  TRSumVariant=Passthrough  SumFdbkVariant=Disabled  SumVariant=Passthrough_P  TsampFilterVariant=InternalTs  TsampNgainVariant=Passthrough  TsampIntegralVariant=Disabled_SignalSpec  ExternalSaturationOutDataTypeStr=Inherit: Same as second input
  P_w : slpidlib/PID Controller  Controller=P  Form=Parallel  TimeDomain=Discrete-time  UseExternalTs=off  SampleTime=-1  IntegratorMethod=Forward Euler  FilterMethod=Forward Euler  ControllerParametersSource=internal  P=1  I=0  D=0  UseFilter=on  N=100  TunerSelectOption=Transfer Function Based (PID Tuner App)  InitialConditionSource=internal  InitialConditionForIntegrator=0  InitialConditionForFilter=0  DifferentiatorICPrevScaledInput=0  ExternalReset=none  TrackingMode=off  Kt=1  LimitOutput=off  SatLimitsSource=internal  UpperSaturationLimit=inf  LowerSaturationLimit=-inf  LinearizeAsGain=off  AntiWindupMode=none  Kb=1  POutMin=[]  POutMax=[]  IOutMin=[]  IOutMax=[]  DOutMin=[]  DOutMax=[]  NOutMin=[]  NOutMax=[]  SumOutMin=[]  SumOutMax=[]  SaturationOutMin=[]  SaturationOutMax=[]  PParamMin=[]  PParamMax=[]  IParamMin=[]  IParamMax=[]  DParamMin=[]  DParamMax=[]  NParamMin=[]  NParamMax=[]  KbParamMin=[]  KbParamMax=[]  KtParamMin=[]  KtParamMax=[]  KbOutMin=[]  KbOutMax=[]  KtOutMin=[]  KtOutMax=[]  IntegratorOutMin=[]  IntegratorOutMax=[]  FilterOutMin=[]  FilterOutMax=[]  SumI1OutMin=[]  SumI1OutMax=[]  SumI2OutMin=[]  SumI2OutMax=[]  SumI3OutMin=[]  SumI3OutMax=[]  SumI4OutMin=[]  SumI4OutMax=[]  SumDOutMin=[]  SumDOutMax=[]  DifferentiatorOutMin=[]  DifferentiatorOutMax=[]  FilterDiffOutCoefMin=[]  FilterDiffOutCoefMax=[]  ReciprocalOutMin=[]  ReciprocalOutMax=[]  SumDenOutMin=[]  SumDenOutMax=[]  SumNumOutMin=[]  SumNumOutMax=[]  DivideOutMin=[]  DivideOutMax=[]  UdiffTsProdOutMin=[]  UdiffTsProdOutMax=[]  NTsProdOutMin=[]  NTsProdOutMax=[]  UintegralTsProdOutMin=[]  UintegralTsProdOutMax=[]  UngainTsProdOutMin=[]  UngainTsProdOutMax=[]  IntegratorContinuousStateAttributes=''  IntegratorStateMustResolveToSignalObject=off  IntegratorRTWStateStorageClass=Auto  FilterContinuousStateAttributes=''  FilterStateMustResolveToSignalObject=off  FilterRTWStateStorageClass=Auto  ParallelPVariant=InternalParameters  IdealPVariant=Disabled  IVariant=Disabled  DVariant=Disabled  IntegratorVariant=Disabled  SatVariant=Disabled  AWVariant=Disabled  PCopyVariant=Disabled  TRVariant=Disabled  FdbkBlocksVariant=Forward  IdealPFdbkVariant=Disabled  SatFdbkVariant=Disabled  DerivativeFilterVariant=Disabled  NVariant=Disabled  NCopyVariant=Disabled_SignalSpec  FilterICVariant=Disabled  IntegratorICVariant=Disabled  ExternalResetVariant=Disabled  TRSumVariant=Passthrough  SumFdbkVariant=Disabled  SumVariant=Passthrough_P  TsampFilterVariant=InternalTs  TsampNgainVariant=Passthrough  TsampIntegralVariant=Disabled_SignalSpec  ExternalSaturationOutDataTypeStr=Inherit: Same as second input
  Selector : Selector  InputPortWidth=3  IndexOptions=Index vector (dialog)  Indices=[1 2]  OutputSizes=1
  Selector1 : Selector  InputPortWidth=3  IndexOptions=Index vector (dialog)  Indices=[2 3 1]  OutputSizes=1
  g : Constant  Value=9.81
  acc_cmd : Outport
  DEBUG : Outport  Port=2
  wires:
  Mux1/1 -> acc_cmd/1
  P_r/1 -> Mux5/3
  Mux6/1 -> Add1/2  "uvw_dot.state"
  Demux/1 -> Mux/1  "u_dot.desired"
  Demux1/2 -> PI_v_dot/1
  Add2/1 -> Mux6/3
  Add3/1 -> Demux3/1  "pqr.error"
  Demux2/3 -> Add2/1
  Add4/1 -> P_w/1  "w.error"
  Demux4/1 -> P_roll/1
  Demux3/2 -> P_q/1
  P_p/1 -> Mux5/1
  Demux/4 -> Mux2/1  "r.desired"
  Demux1/3 -> PI_w_dot/1
  Selector/1 -> Gain/1
  g/1 -> Add2/2
  Demux/2 -> Mux/2  "v_dot.desired"
  P_w/1 -> Mux/3  "w_dot"
  Selector1/1 -> Add3/1  "pqr.desired"
  Mux2/1 -> Selector1/1
  Mux4/1 -> Mux1/1
  Demux2/1 -> Mux6/1
  Demux3/3 -> P_r/1
  z_vel/1 -> Add4/2  "w.state"
  Demux3/1 -> P_p/1
  PI_w_dot/1 -> Mux4/3
  P_q/1 -> Mux5/2
  gyro/1 -> Add3/2  "pqr.state"
  euler/1 -> Selector/1  "pitchroll.state"
  PI_u_dot/1 -> Mux4/1
  PI_v_dot/1 -> Mux4/2
  Demux2/2 -> Mux6/2
  Mux/1 -> Add1/1  "uvw_dot.desired"
  RC/1 -> Demux/1
  Mux5/1 -> Mux1/2, DEBUG/1
  Gain/1 -> Demux4/1  "pitchroll.error"
  Add1/1 -> Demux1/1  "uvw_dot.error"
  acc/1 -> Demux2/1  "m/s²"
  Demux/3 -> Add4/1  "w.desired"
  Demux4/2 -> P_pitch/1
  P_roll/1 -> Mux3/1
  Demux1/1 -> PI_u_dot/1
  Mux3/1 -> Mux2/2  "pq.desired"
  P_pitch/1 -> Mux3/2

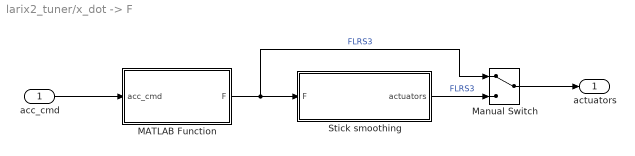
== system larix2_tuner/x_dot -> F ==
  acc_cmd : Inport
  MATLAB Function : MATLAB Function  TreatAsAtomicUnit=on
  Manual Switch : ManualSwitch
  Stick smoothing : Subsystem
  actuators : Outport  OutDataTypeStr=double
  wires:
  Stick smoothing/1(actuators) -> Manual Switch/2  "FLRS3"
  acc_cmd/1 -> MATLAB Function/1(acc_cmd)
  MATLAB Function/1(F) -> Manual Switch/1, Stick smoothing/1(F)  "FLRS3"
  Manual Switch/1 -> actuators/1

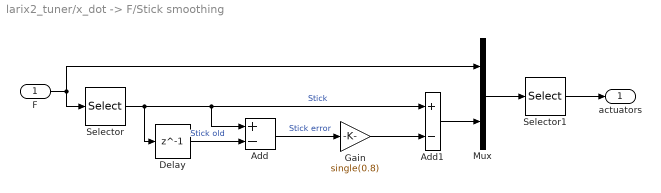
== system larix2_tuner/x_dot -> F/Stick smoothing ==
  F : Inport
  Add : Sum  Inputs=+-
  Add1 : Sum  Inputs=+-
  Delay : Delay  DelayLength=1
  Gain : Gain  Gain=single(0.8)
  Mux : Mux  Inputs=2
  Selector : Selector  InputPortWidth=4  IndexOptions=Index vector (dialog)  Indices=[3]  OutputSizes=1
  Selector1 : Selector  InputPortWidth=5  IndexOptions=Index vector (dialog)  Indices=[1 2 5 4]  OutputSizes=1
  actuators : Outport
  wires:
  F/1 -> Mux/1, Selector/1
  Selector/1 -> Add/1, Add1/1, Delay/1  "Stick"
  Delay/1 -> Add/2  "Stick old"
  Mux/1 -> Selector1/1
  Selector1/1 -> actuators/1
  Add/1 -> Gain/1  "Stick error"
  Add1/1 -> Mux/2
  Gain/1 -> Add1/2

== matlab function larix2_tuner/Dynamics Model/Dynamics ==
  data: F input; x_dotdot output; e input; x_dot input
function x_dotdot = fcn(F,e,x_dot)


F1 = F(1);
F2 = F(2);
stick = F(3);
F3 = F(4);


e0 = e(1);
e1 = e(2);
e2 = e(3);
e3 = e(4);

u = x_dot(1);
v = x_dot(2);
w = x_dot(3);
p = x_dot(4);
q = x_dot(5);
r = x_dot(6);

%}

g = -9.81;
rho_air = 1.225; 
eta_air = 1.802e-5;

nu_hull =  1;
nu_fin = 0.6;

blimp = inertias();
prp = blimp.prp;
par = blimp.par;
in = blimp.mM;


H = prp.mass_H;
W = in.mass*g;
B = H*g - W;

V_ref = prp.volume_blimp_body; %volume based on two semi ellipsoids
S_ref = V_ref^(2/3);
L_ref = V_ref^(1/3);

mx = in.M(1,1);
my = in.M(2,2);
mz = in.M(3,3);

Jxx = in.M(4,4);
Jyy = in.M(5,5);
Jzz = in.M(6,6);
Jxz = in.M(3,6);
 
%DYNAMICS

f1 = -mz*w*q + my*r*v + in.mass*(in.a(1)*( q^2 + r^2) - in.a(3)*r*p);
f2 = -mx*u*r + mz*p*w + in.mass*(-in.a(1)*p*q - in.a(3)*r*q);
f3 = -my*v*p + mx*q*u + in.mass*(-in.a(1)*r*p + in.a(3)*(q^2 + p^2));
f4 = -(Jzz - Jyy)*r*q + Jxz*p*q + in.mass*in.a(3)*(u*r - p*w);
f5 = -(Jxx - Jzz)*p*r + Jxz*(r^2 - p^2) + in.mass*(in.a(1)*(v*p - q*u) - in.a(3)*(w*q - r*v));
f6 = -(Jyy - Jxx)*q*p - Jxz*q*r + in.mass*(-in.a(1)*(u*r - p*w));


F = [f1; f2; f3; f4; f5; f6];

%GRAVITATIONAL FORCES

DCM = [e0^2+e1^2-e2^2-e3^2, 2*(e1*e2-e0*e3),2*(e0*e2-e1*e3);...
        2*(e0*e3-e1*e2),e0^2-e1^2+e2^2-e3^2,2*(e2*e3-e0*e1);...
        2*(e1*e3-e0*e2),2*(e0*e1-e2*e3),e0^2-e1^2-e2^2+e3^2];


    
G = [DCM(3,1)*(W+B); DCM(3,2)*(W+B); DCM(3,3)*(W+B);-DCM(3,2)*in.a(3)*W; (DCM(3,1)*in.a(3)-DCM(3,3)*in.a(1))*W; DCM(3,2)*in.a(1)*W];


%PROPULSION FORCES


Pu = (F1+F2)*sin(stick*pi/2);
Pv = F3;
Pw = (F1+F2)*cos(stick*pi/2);

Pp = (F1-F2)*sin(stick*pi/2)*prp.length_stick-F3*par.bot_rud_motor.position(3);
Pq_v = cross([Pu 0 Pw],(par.stick.position-in.CG));
Pq = Pq_v(2);
Pr = (-F1+F2)*prp.length_stick*sin(stick*pi/2)+F3*par.bot_rud_motor.position(3);

P = [Pu; Pv; Pw; Pp; Pq; Pr];

% AERO FORCES


fh = (prp.length_tip_to_fin - prp.length_blimp_a1)/prp.length_blimp_a2;
xcv = prp.length_blimp_a1-(4*pi/3)*(prp.length_blimp_a1-prp.length_blimp_a2);

I_1 = pi*((prp.radius_blimp_body^2)/S_ref)*(1-fh^2);
I_3 = pi*((prp.radius_blimp_body^2)/(3*prp.length_blimp_body*S_ref)*(prp.length_blimp_a1 - 2*prp.length_blimp_a2*(fh^3) - 3*prp.length_blimp_a1*(fh^2)) - xcv*I_1/prp.length_blimp_body);


J_1 = prp.radius_blimp_body/(2*S_ref)*(pi*prp.length_blimp_a1 + prp.length_blimp_a2*sqrt(1-fh*fh)*fh + 2*prp.length_blimp_a2*asin(fh));
J_2 = (J_1/prp.length_blimp_body)*(prp.length_blimp_a1-xcv) + (2*prp.radius_blimp_body/(3*prp.length_blimp_body*S_ref))*(prp.length_blimp_a2^2 - prp.length_blimp_a1^2 - (prp.length_blimp_a2^2)*(1-fh^2)^(3/2));

Re = prp.length_tip_to_fin*rho_air/eta_air;
Cf = 0.045*Re^(-1/6);

Cdchull = 1.17;     %Cd of cylinder in transverse flow
Cdcfin = 1.28;       %Cd of Plate in transverse flow

%Cdcross = -(1/S_ref)*(Cdchull*J_1*S_ref+Cdcfin*S_fin);

S_fin = 0.32;
lf1 = 3.84;          %platzhalter abstand cv zu aero center fin
lf2 = 3.9;
lf3 = 1.65/2;


Cx1 = Cf*(4*(prp.length_blimp_body/prp.radius_blimp_body)^(1/3)+6*(prp.length_blimp_body/prp.radius_blimp_body)^(-1.2)+24*(prp.length_blimp_body/prp.radius_blimp_body)^(-2.7)); %Cd0H        KTh paper       cgcl_xial Cd & b as mcgcl_x_diameter/2 
Cx2 = (in.k(2)-in.k(1))*nu_hull*I_1*S_ref;             %munk lift
Cx3 = 0;

Cy1 = -Cx2;                                       %dCl/da = 2*pi
Cy2 = -pi*2*S_fin*nu_fin;
Cy3 = -(Cdchull*J_1*S_ref+Cdcfin*2*S_fin);

Cz1 = -Cy1;
Cz2 = Cy2;
Cz3 = Cy3;          %only if aero influence of gondola is negelected;

Cl3= -Cdcfin*2*S_fin*lf3*4;

Cm1 = -(in.k(1)-in.k(2))*nu_hull*I_3*S_ref*prp.length_blimp_body;
Cm2 = -pi*S_fin*nu_fin*lf1;
Cm3 = -(Cdchull*J_2*S_ref*prp.length_blimp_body+Cdcfin*2*S_fin*lf2);
Cm5 = -Cdcfin*S_fin*2*lf2*prp.length_blimp_body*prp.length_blimp_body;

Cn1 = Cm1;
Cn2 = Cm2;

Cn3 = Cm3;
Cn5 = -(Cdcfin*2*S_fin*lf2*prp.length_blimp_body*prp.length_blimp_body);

Cm5 = 0;
Cn5 = 0;
U_abs = sqrt(u^2 +v^2 +w^2);



if u == 0
    a = 0;
else
    a = atan(w/u);
end
if U_abs == 0
    b = 0;
else
    b = asin(v/U_abs);
end
    
    
e = sqrt(((prp.length_blimp_body*0.5)*(prp.length_blimp_body*0.5)-prp.radius_blimp_body*prp.radius_blimp_body)/(prp.length_blimp_body*0.5));

S = pi*prp.radius_blimp_body*(prp.radius_blimp_body+(prp.length_blimp_body*0.5)*(prp.length_blimp_body*0.5)*sin(e)/e);

X = 0.5*rho_air*(U_abs^2)*(Cx1*(cos(a)^2)*(cos(b)^2) + Cx2*sin(2*a)*sin(a/2));
Y = 0.5*rho_air*(U_abs^2)*(Cy1*cos(b/2)*sin(2*b)+Cy2*sin(2*b) + Cy3*sin(b)*sin(abs(b)));
Z = 0.5*rho_air*(U_abs^2)*(Cz1*cos(a/2)*sin(2*a)+Cz2*sin(2*a) + Cz3*sin(a)*sin(abs(a)));

L = 0.5*rho_air*(U_abs^2)*(0.5*rho_air*S*Cl3*p*abs(p));
M = 0.5*rho_air*(U_abs^2)*(Cm1*cos(a/2)*sin(2*a)+Cm2*sin(2*a)+Cm3*sin(a)*sin(abs(a))+0.5*rho_air*S*Cm5*q*abs(q));
N = 0.5*rho_air*(U_abs^2)*(Cn1*cos(b/2)*sin(2*b)+Cn2*sin(2*b)+Cn3*sin(b)*sin(abs(b))+0.5*rho_air*S*Cn5*r*abs(r));

%prp.length_blimp_body*S*
A = [X;Y;Z;L;M;N];


x_dotdot = in.M\(A + F + G + P);
end

== matlab function larix2_tuner/x_dot -> F/MATLAB Function ==
  data: acc_cmd input; F output size=4; blimp parameter
function F = fcn(acc_cmd, blimp)
H = blimp.prp.mass_H;

lPVH = blimp.par.stick.position(1) - blimp.par.bot_rud_motor.position(1);   %distance between front and back props

lPLR = blimp.prp.length_stick;            %distance between Prop L and R
lCGV = blimp.par.stick.position(1);             %distance from front props to cg


F3_min = -0.11*9.81; %[kg]
F3_max = 0.035*9.81; %[kg]




u_dot = acc_cmd(1);
v_dot = acc_cmd(2);
w_dot = acc_cmd(3);
p_dot = acc_cmd(4);
q_dot = acc_cmd(5);
r_dot = acc_cmd(6);

stick = u_dot/(0.5*9.81);

FLRuw = H*w_dot/(cos(stick*pi/2));

FLRq = lCGV*q_dot;

FLRp = p_dot*lPLR/2;

if stick == 0
    delta_Fv = 0;
    F3v = 0;
else
if v_dot >0 
    delta_Fv = abs(stick)*lPVH*min(F3_max,v_dot*H)/(sin(stick*pi/2)*lPLR);
    F3v = abs(stick)*min(F3_max,v_dot*H);
else
    delta_Fv = abs(stick)*lPVH*max(F3_min,v_dot*H)/(sin(stick*pi/2)*lPLR);
    F3v = abs(stick)*max(F3_min,v_dot*H);
end
end

FL = FLRuw + FLRq + delta_Fv + FLRp;
FR = FLRuw + FLRq - delta_Fv - FLRp;


F3r = 0.8*r_dot;


F3 = F3r + F3v;



LRS3 = [FL FR stick F3];

F = LRS3(1,:)';
